simulink model "settling_time"  (R2023b)
settings: Solver=VariableStepAuto  StartTime=0.0  StopTime=10.0  MaxStep=Ts * 0.001  MinStep=Ts * 0.0001  RelTol=1e-3
values from neighbouring files (symbols this model uses):
  Ts = 5e-3    (= 0.005)    [algebraic_2019_06.m]
libraries: cstblocks x3
settings Model: Creator=lucapili  LastModifiedBy=lucap

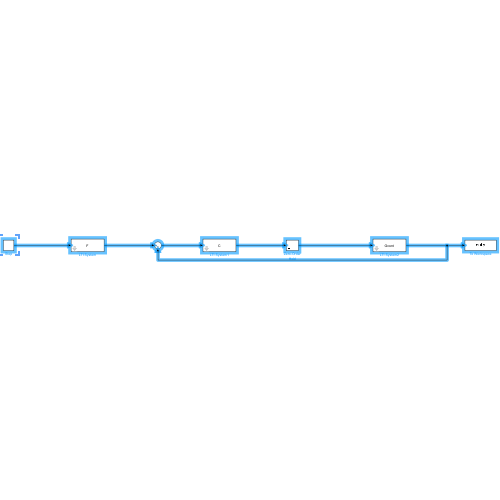
[thumbnail: Simulink's stored preview of the top-level diagram]
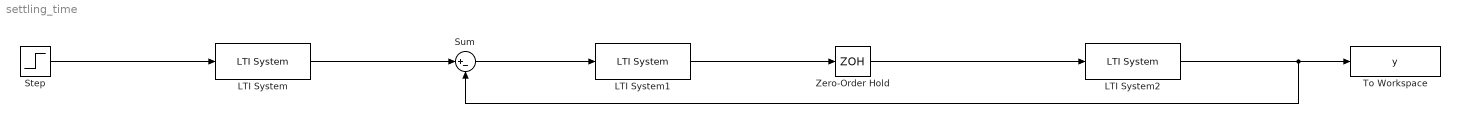
== system settling_time ==
  LTI System : cstblocks/LTI System  sys=F  IC=[]  PadeOrder=0
  LTI System1 : cstblocks/LTI System  sys=C  IC=[]  PadeOrder=0
  LTI System2 : cstblocks/LTI System  sys=Gcont  IC=[]  PadeOrder=0
  Step : Step  Time=0  SampleTime=0
  Sum : Sum  Inputs=|+-
  To Workspace : ToWorkspace  VariableName=y  SaveFormat=Timeseries  SampleTime=Ts * 0.001
  Zero-Order Hold : ZeroOrderHold  SampleTime=Ts
  wires:
  Step/1 -> LTI System/1
  LTI System/1 -> Sum/1
  Sum/1 -> LTI System1/1
  LTI System1/1 -> Zero-Order Hold/1
  Zero-Order Hold/1 -> LTI System2/1
  LTI System2/1 -> Sum/2, To Workspace/1
